simulink model "model_mamdani"  (R2016a)
settings: Solver=FixedStepAuto  StartTime=0.0  StopTime=1000  FixedStep=1  RelTol=1e-3
values from neighbouring files (symbols this model uses):
  a = 1    [prob_init.m]
  b = 2    [prob_init.m]
  c = 1    [prob_init.m]
  g = 9.8    [prob_init.m]
libraries: fuzblock x1
settings Model: Creator=Leonor  LastModifiedBy=Leonor
settings DebuggingCC: MaxConsecutiveZCsMsg=none

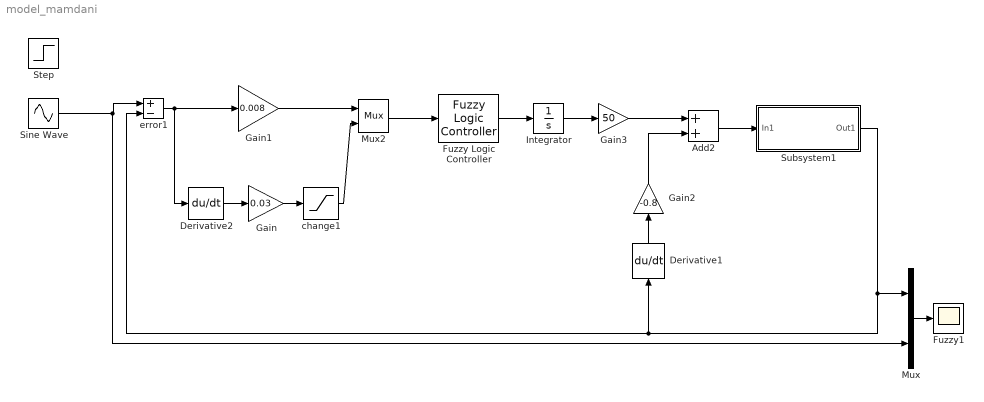
== system model_mamdani ==
  Add2 : Sum
  Derivative1 : Derivative
  Derivative2 : Derivative
  Fuzzy Logic Controller : fuzblock/Fuzzy Logic  Controller  fis=fis
  Fuzzy1 : Scope
  Gain : Gain  Gain=0.03
  Gain1 : Gain  Gain=0.008
  Gain2 : Gain  Gain=-0.8
  Gain3 : Gain  Gain=50
  Integrator : Integrator
  Mux : Mux  Inputs=2
  Mux2 : Mux  Inputs=2
  Sine Wave : Sin  Bias=2  Frequency=2*pi/1000  SampleTime=0
  Step : Step  Time=2  Before=1  After=2  SampleTime=0
  Subsystem1 : Subsystem
  change1 : Saturate  UpperLimit=5  LowerLimit=-5  ZeroCross=off
  error1 : Sum  Inputs=+-  SaturateOnIntegerOverflow=on  InputSameDT=on  OutDataTypeStr=Inherit: Same as first input
  wires:
  Mux2/1 -> Fuzzy Logic Controller/1
  Sine Wave/1 -> error1/1, Mux/2
  Derivative2/1 -> Gain/1
  Fuzzy Logic Controller/1 -> Integrator/1
  Mux/1 -> Fuzzy1/1
  error1/1 -> Derivative2/1, Gain1/1
  Gain1/1 -> Mux2/1
  Derivative1/1 -> Gain2/1
  Subsystem1/1("Out1 ") -> Mux/1, error1/2, Derivative1/1
  Integrator/1 -> Gain3/1
  Gain3/1 -> Add2/1
  Gain/1 -> change1/1
  change1/1 -> Mux2/2
  Add2/1 -> Subsystem1/1(In1)
  Gain2/1 -> Add2/2

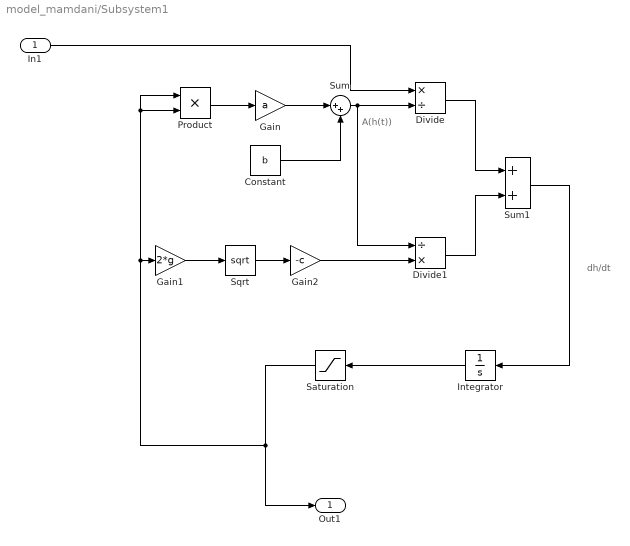
== system model_mamdani/Subsystem1 ==
  note: dh/dt
  note: A(h(t))
  In1 : Inport
  Constant : Constant  Value=b
  Divide : Product  Inputs=*/
  Divide1 : Product  Inputs=/*
  Gain : Gain  Gain=a
  Gain1 : Gain  Gain=2*g
  Gain2 : Gain  Gain=-c
  Integrator : Integrator  InitialCondition=1
  Product : Product
  Saturation : Saturate  UpperLimit=5  LowerLimit=1
  Sqrt : Sqrt  SaturateOnIntegerOverflow=on
  Sum : Sum  Inputs=|++
  Sum1 : Sum
  "Out1 " : Outport
  wires:
  Product/1 -> Gain/1
  Gain/1 -> Sum/1
  Constant/1 -> Sum/2
  Sum/1 -> Divide/2, Divide1/1
  Gain1/1 -> Sqrt/1
  Sqrt/1 -> Gain2/1
  Gain2/1 -> Divide1/2
  Divide/1 -> Sum1/1
  Divide1/1 -> Sum1/2
  Sum1/1 -> Integrator/1
  Integrator/1 -> Saturation/1
  Saturation/1 -> "Out1 "/1, Product/2, Product/1, Gain1/1
  In1/1 -> Divide/1
